simulink model "VFlexP"  (R2025a)
settings: Solver=ode23tb  StartTime=0.0  StopTime=40  FixedStep=5e-5
model workspace (MAT data in the model file):
  DCop_DCBUCK.op = opcond.OperatingPoint
  DCop_DCBUCK.op.Model_ = 'untitled4'
  DCop_DCBUCK.op.States_(1) = opcond.StatePoint
  DCop_DCBUCK.op.States_(1).Nx_ = 1
  DCop_DCBUCK.op.States_(1).Block_ = 'untitled4/DCBUCK/Integrator'
  DCop_DCBUCK.op.States_(1).x_ = 0.0993111458289
  DCop_DCBUCK.op.States_(2) = opcond.StatePoint
  DCop_DCBUCK.op.States_(2).Nx_ = 1
  DCop_DCBUCK.op.States_(2).Block_ = 'untitled4/DCBUCK/Integrator1'
  DCop_DCBUCK.op.States_(2).x_ = -1.0059432275
  DCop_DCBUCK.op_report = opcond.OperatingReport
  DCop_DCBUCK.op_report.Outputs_ = opcond.OutputReport
  DCop_DCBUCK.op_report.Outputs_.yspec_ = 0.0993111426985
  DCop_DCBUCK.op_report.Outputs_.Block_ = 'untitled4/out_trim1'
  DCop_DCBUCK.op_report.Outputs_.PortWidth_ = 1
  DCop_DCBUCK.op_report.Outputs_.PortNumber_ = NaN
  DCop_DCBUCK.op_report.Outputs_.y_ = 0.0993111458289
  DCop_DCBUCK.op_report.Outputs_.Known_ = 1
  DCop_DCBUCK.op_report.Outputs_.Min_ = -Inf
  DCop_DCBUCK.op_report.Outputs_.Max_ = Inf
  DCop_DCBUCK.op_report.TerminationString_ = 'Operating point specifications were successfully met.'
  DCop_DCBUCK.op_report.OptimizationOutput_.iterations = 1
  DCop_DCBUCK.op_report.OptimizationOutput_.funcCount = 6
  DCop_DCBUCK.op_report.OptimizationOutput_.constrviolation = 8.64996069397e-05
  DCop_DCBUCK.op_report.OptimizationOutput_.stepsize = 2.19887440386
  DCop_DCBUCK.op_report.OptimizationOutput_.algorithm = 'interior-point'
  DCop_DCBUCK.op_report.OptimizationOutput_.firstorderopt = 0
  DCop_DCBUCK.op_report.OptimizationOutput_.cgiterations = 0
  DCop_DCBUCK.op_report.OptimizationOutput_.message = 'Local minimum found that satisfies the constraints.
    | 
    | Optimization completed because the objective function is non-decreasing in 
    | feasible directions, to within the value of the optimality tolerance,
    | and constraints are satisfied to within the value of the constraint tolerance.
    | 
    | <stopping criteria details>
    | 
    | Optimization completed: The relative first-order optimality measure, 0.000000e+00,
    | is less than options.OptimalityTolerance = 1.000000e-06, and the relative maximum constraint
    | violation, 9.451558e-09, is less than options.ConstraintTolerance = 1.000000e-06.'
  DCop_DCBUCK.op_report.OptimizationOutput_.bestfeasible = []
  DCop_DCBUCK.op_report.Model_ = 'untitled4'
  DCop_DCBUCK.op_report.States_(1) = opcond.StateReport
  DCop_DCBUCK.op_report.States_(1).dx_ = 8.64996069397e-05
  DCop_DCBUCK.op_report.States_(1).Nx_ = 1
  DCop_DCBUCK.op_report.States_(1).Block_ = 'untitled4/DCBUCK/Integrator'
  DCop_DCBUCK.op_report.States_(1).x_ = 0.0993111458289
  DCop_DCBUCK.op_report.States_(1).SteadyState_ = 1
  DCop_DCBUCK.op_report.States_(1).dxMin_ = -Inf
  DCop_DCBUCK.op_report.States_(1).dxMax_ = Inf
  DCop_DCBUCK.op_report.States_(1).Known_ = 0
  DCop_DCBUCK.op_report.States_(1).Min_ = -Inf
  DCop_DCBUCK.op_report.States_(1).Max_ = Inf
  DCop_DCBUCK.op_report.States_(2) = opcond.StateReport
  DCop_DCBUCK.op_report.States_(2).dx_ = -1.77018447944e-06
  DCop_DCBUCK.op_report.States_(2).Nx_ = 1
  DCop_DCBUCK.op_report.States_(2).Block_ = 'untitled4/DCBUCK/Integrator1'
  DCop_DCBUCK.op_report.States_(2).x_ = -1.0059432275
  DCop_DCBUCK.op_report.States_(2).SteadyState_ = 1
  DCop_DCBUCK.op_report.States_(2).dxMin_ = -Inf
  DCop_DCBUCK.op_report.States_(2).dxMax_ = Inf
  DCop_DCBUCK.op_report.States_(2).Known_ = 0
  DCop_DCBUCK.op_report.States_(2).Min_ = -Inf
  DCop_DCBUCK.op_report.States_(2).Max_ = Inf
  Grid_CCVSC_idx = [2; 3; 4; 5; 6; 7; 8; 9; 10; 11; 12]
  Grid_CCVSCs = 1
  Grid_CCVSCs_buses = 1
  Grid_CCVSCs_toM = [0 1 0 0 0 0 0 0 0 0 0 0 ... (781 elements, 71x11)]
  Grid_C_Lines = [0.1 0.1 0.1 0.1]
  Grid_Cbuses = [0.05000002 0.10000002 0.10000002 0.10000002 0.05000002]
  Grid_DC.include = 1
  Grid_DC.Nbuses = 3
  Grid_DC.from = [1; 2]
  Grid_DC.to = [2; 3]
  Grid_DC.bus = [3; 4; 5]
  Grid_DC.v = [0.9920000006 0.9960000002 1]
  Grid_DC.Lines_toM : sparse (value not decoded)
  Grid_DC.Lines_fromM : sparse (value not decoded)
  Grid_DC.R_Lines = [0.01 0.01]
  Grid_DC.L_Lines = [0 0]
  Grid_DC.CbusDC = [0.0001; 0.0001; 0.0001]
  Grid_DC.i_branch = [-0.39999996  -0.39999996; -0.39999998  -0.39999998]
  Grid_DC.Rbus = [50000000; 50000000; 50000000]
  Grid_DC.DC_CCVSCs_toM = [0  0; 1  0; 0  0; 0  1; 0  0]
  Grid_DC.DC_CCVSCs_DC_toM = [1  0; 0  0; 0  1]
  Grid_DC.DC_CCVSCs_buses = [2; 4]
  Grid_DC.DC_CCVSCs_DC_buses = [1; 3]
  Grid_DC.DC_CCVSC_dparams.ratio = [1 1]
  Grid_DC.DC_CCVSC_dparams.type = [1 2]
  Grid_DC.DC_CCVSC_dparams.Rf = [0.0001 0.0002]
  Grid_DC.DC_CCVSC_dparams.Lf = [0.15 0.35]
  Grid_DC.DC_CCVSC_dparams.alpha1 = [0.0001 0.0001]
  Grid_DC.DC_CCVSC_dparams.alpha2 = [0.015 0.015]
  Grid_DC.DC_CCVSC_dparams.alpha3 = [0.2 0.02]
  Grid_DC.DC_CCVSC_dparams.Gsw = [0 0]
  Grid_DCop_DCBUCK.op = opcond.OperatingPoint
  Grid_DCop_DCBUCK.op.Model_ = 'untitled'
  Grid_DCop_DCBUCK.op.States_(1) = opcond.StatePoint
  Grid_DCop_DCBUCK.op.States_(1).Nx_ = 1
  Grid_DCop_DCBUCK.op.States_(1).Block_ = 'untitled/DCBUCK/Integrator'
  Grid_DCop_DCBUCK.op.States_(1).x_ = 0.297042066445
  Grid_DCop_DCBUCK.op.States_(2) = opcond.StatePoint
  Grid_DCop_DCBUCK.op.States_(2).Nx_ = 1
  Grid_DCop_DCBUCK.op.States_(2).Block_ = 'untitled/DCBUCK/Integrator1'
  Grid_DCop_DCBUCK.op.States_(2).x_ = -1.00698752155
  Grid_DCop_DCBUCK.op_report = opcond.OperatingReport
  Grid_DCop_DCBUCK.op_report.Outputs_ = opcond.OutputReport
  Grid_DCop_DCBUCK.op_report.Outputs_.yspec_ = 0.297042068743
  Grid_DCop_DCBUCK.op_report.Outputs_.Block_ = 'untitled/out_trim1'
  Grid_DCop_DCBUCK.op_report.Outputs_.PortWidth_ = 1
  Grid_DCop_DCBUCK.op_report.Outputs_.PortNumber_ = NaN
  Grid_DCop_DCBUCK.op_report.Outputs_.y_ = 0.297042066445
  Grid_DCop_DCBUCK.op_report.Outputs_.Known_ = 1
  Grid_DCop_DCBUCK.op_report.Outputs_.Min_ = -Inf
  Grid_DCop_DCBUCK.op_report.Outputs_.Max_ = Inf
  Grid_DCop_DCBUCK.op_report.TerminationString_ = 'Operating point specifications were successfully met.'
  Grid_DCop_DCBUCK.op_report.OptimizationOutput_.iterations = 1
  Grid_DCop_DCBUCK.op_report.OptimizationOutput_.funcCount = 6
  Grid_DCop_DCBUCK.op_report.OptimizationOutput_.constrviolation = 8.27288844959e-05
  Grid_DCop_DCBUCK.op_report.OptimizationOutput_.stepsize = 2.12653445023
  Grid_DCop_DCBUCK.op_report.OptimizationOutput_.algorithm = 'interior-point'
  Grid_DCop_DCBUCK.op_report.OptimizationOutput_.firstorderopt = 0
  Grid_DCop_DCBUCK.op_report.OptimizationOutput_.cgiterations = 0
  Grid_DCop_DCBUCK.op_report.OptimizationOutput_.message = 'Local minimum found that satisfies the constraints.
    | 
    | Optimization completed because the objective function is non-decreasing in 
    | feasible directions, to within the value of the optimality tolerance,
    | and constraints are satisfied to within the value of the constraint tolerance.
    | 
    | <stopping criteria details>
    | 
    | Optimization completed: The relative first-order optimality measure, 0.000000e+00,
    | is less than options.OptimalityTolerance = 1.000000e-06, and the relative maximum constraint
    | violation, 8.342696e-09, is less than options.ConstraintTolerance = 1.000000e-06.'
  Grid_DCop_DCBUCK.op_report.OptimizationOutput_.bestfeasible = []
  Grid_DCop_DCBUCK.op_report.Model_ = 'untitled'
  Grid_DCop_DCBUCK.op_report.States_(1) = opcond.StateReport
  Grid_DCop_DCBUCK.op_report.States_(1).dx_ = 8.27288844959e-05
  Grid_DCop_DCBUCK.op_report.States_(1).Nx_ = 1
  Grid_DCop_DCBUCK.op_report.States_(1).Block_ = 'untitled/DCBUCK/Integrator'
  Grid_DCop_DCBUCK.op_report.States_(1).x_ = 0.297042066445
  Grid_DCop_DCBUCK.op_report.States_(1).SteadyState_ = 1
  Grid_DCop_DCBUCK.op_report.States_(1).dxMin_ = -Inf
  Grid_DCop_DCBUCK.op_report.States_(1).dxMax_ = Inf
  Grid_DCop_DCBUCK.op_report.States_(1).Known_ = 0
  Grid_DCop_DCBUCK.op_report.States_(1).Min_ = -Inf
  Grid_DCop_DCBUCK.op_report.States_(1).Max_ = Inf
  Grid_DCop_DCBUCK.op_report.States_(2) = opcond.StateReport
  Grid_DCop_DCBUCK.op_report.States_(2).dx_ = 1.29998784019e-06
  Grid_DCop_DCBUCK.op_report.States_(2).Nx_ = 1
  Grid_DCop_DCBUCK.op_report.States_(2).Block_ = 'untitled/DCBUCK/Integrator1'
  Grid_DCop_DCBUCK.op_report.States_(2).x_ = -1.00698752155
  Grid_DCop_DCBUCK.op_report.States_(2).SteadyState_ = 1
  Grid_DCop_DCBUCK.op_report.States_(2).dxMin_ = -Inf
  Grid_DCop_DCBUCK.op_report.States_(2).dxMax_ = Inf
  Grid_DCop_DCBUCK.op_report.States_(2).Known_ = 0
  Grid_DCop_DCBUCK.op_report.States_(2).Min_ = -Inf
  Grid_DCop_DCBUCK.op_report.States_(2).Max_ = Inf
  Grid_DCop_DC_PES.op = opcond.OperatingPoint
  Grid_DCop_DC_PES.op.Model_ = 'untitled'
  Grid_DCop_DC_PES.op.States_(1) = opcond.StatePoint
  Grid_DCop_DC_PES.op.States_(1).Nx_ = 1
  Grid_DCop_DC_PES.op.States_(1).Block_ = 'untitled/DC_PES/Integrator'
  Grid_DCop_DC_PES.op.States_(1).x_ = 0.0833333466671
  Grid_DCop_DC_PES.op.States_(2) = opcond.StatePoint
  Grid_DCop_DC_PES.op.States_(2).Nx_ = 1
  Grid_DCop_DC_PES.op.States_(2).Block_ = 'untitled/DC_PES/Integrator1'
  Grid_DCop_DC_PES.op.States_(2).x_ = 0.166666684167
  Grid_DCop_DC_PES.op.States_(3) = opcond.StatePoint
  Grid_DCop_DC_PES.op.States_(3).Nx_ = 1
  Grid_DCop_DC_PES.op.States_(3).Block_ = 'untitled/DC_PES/Integrator2'
  Grid_DCop_DC_PES.op.States_(3).x_ = 0.0833333466671
  Grid_DCop_DC_PES.op.States_(4) = opcond.StatePoint
  Grid_DCop_DC_PES.op.States_(4).Nx_ = 1
  Grid_DCop_DC_PES.op.States_(4).Block_ = 'untitled/DC_PES/WOF_d/I'
  Grid_DCop_DC_PES.op.States_(4).x_ = 9.16666653332e-13
  Grid_DCop_DC_PES.op_report = opcond.OperatingReport
  Grid_DCop_DC_PES.op_report.Outputs_ = opcond.OutputReport
  Grid_DCop_DC_PES.op_report.Outputs_.yspec_ = 0.166666666667
  Grid_DCop_DC_PES.op_report.Outputs_.Block_ = 'untitled/out_trim1'
  Grid_DCop_DC_PES.op_report.Outputs_.PortWidth_ = 1
  Grid_DCop_DC_PES.op_report.Outputs_.PortNumber_ = NaN
  Grid_DCop_DC_PES.op_report.Outputs_.y_ = 0.166666684167
  Grid_DCop_DC_PES.op_report.Outputs_.Known_ = 1
  Grid_DCop_DC_PES.op_report.Outputs_.Min_ = -Inf
  Grid_DCop_DC_PES.op_report.Outputs_.Max_ = Inf
  Grid_DCop_DC_PES.op_report.TerminationString_ = 'Operating point specifications were successfully met.'
  Grid_DCop_DC_PES.op_report.OptimizationOutput_.iterations = 1
  Grid_DCop_DC_PES.op_report.OptimizationOutput_.funcCount = 10
  Grid_DCop_DC_PES.op_report.OptimizationOutput_.constrviolation = 1.74999997271e-08
  Grid_DCop_DC_PES.op_report.OptimizationOutput_.stepsize = 1.54110347542
  Grid_DCop_DC_PES.op_report.OptimizationOutput_.algorithm = 'interior-point'
  Grid_DCop_DC_PES.op_report.OptimizationOutput_.firstorderopt = 0
  Grid_DCop_DC_PES.op_report.OptimizationOutput_.cgiterations = 0
  Grid_DCop_DC_PES.op_report.OptimizationOutput_.message = 'Local minimum found that satisfies the constraints.
    | 
    | Optimization completed because the objective function is non-decreasing in 
    | feasible directions, to within the value of the optimality tolerance,
    | and constraints are satisfied to within the value of the constraint tolerance.
    | 
    | <stopping criteria details>
    | 
    | Optimization completed: The relative first-order optimality measure, 0.000000e+00,
    | is less than options.OptimalityTolerance = 1.000000e-06, and the relative maximum constraint
    | violation, 1.750000e-08, is less than options.ConstraintTolerance = 1.000000e-06.'
  Grid_DCop_DC_PES.op_report.OptimizationOutput_.bestfeasible.x = [0.166666684167; 9.16666653332e-13; 0.0833333466671; 0.0833333466671]
  Grid_DCop_DC_PES.op_report.OptimizationOutput_.bestfeasible.fval = 0
  Grid_DCop_DC_PES.op_report.OptimizationOutput_.bestfeasible.constrviolation = 1.74999997271e-08
  Grid_DCop_DC_PES.op_report.OptimizationOutput_.bestfeasible.firstorderopt = 0
  Grid_DCop_DC_PES.op_report.Model_ = 'untitled'
  Grid_DCop_DC_PES.op_report.States_(1) = opcond.StateReport
  Grid_DCop_DC_PES.op_report.States_(1).Nx_ = 1
  Grid_DCop_DC_PES.op_report.States_(1).Block_ = 'untitled/DC_PES/Integrator'
  Grid_DCop_DC_PES.op_report.States_(1).x_ = 0.0833333466671
  Grid_DCop_DC_PES.op_report.States_(1).SteadyState_ = 1
  Grid_DCop_DC_PES.op_report.States_(1).dxMin_ = -Inf
  Grid_DCop_DC_PES.op_report.States_(1).dxMax_ = Inf
  Grid_DCop_DC_PES.op_report.States_(1).Known_ = 0
  Grid_DCop_DC_PES.op_report.States_(1).Min_ = -Inf
  Grid_DCop_DC_PES.op_report.States_(1).Max_ = Inf
  Grid_DCop_DC_PES.op_report.States_(2) = opcond.StateReport
  Grid_DCop_DC_PES.op_report.States_(2).dx_ = 9.16666659245e-09
  Grid_DCop_DC_PES.op_report.States_(2).Nx_ = 1
  Grid_DCop_DC_PES.op_report.States_(2).Block_ = 'untitled/DC_PES/Integrator1'
  Grid_DCop_DC_PES.op_report.States_(2).x_ = 0.166666684167
  Grid_DCop_DC_PES.op_report.States_(2).SteadyState_ = 1
  Grid_DCop_DC_PES.op_report.States_(2).dxMin_ = -Inf
  Grid_DCop_DC_PES.op_report.States_(2).dxMax_ = Inf
  Grid_DCop_DC_PES.op_report.States_(2).Known_ = 0
  Grid_DCop_DC_PES.op_report.States_(2).Min_ = -Inf
  Grid_DCop_DC_PES.op_report.States_(2).Max_ = Inf
  Grid_DCop_DC_PES.op_report.States_(3) = opcond.StateReport
  Grid_DCop_DC_PES.op_report.States_(3).Nx_ = 1
  Grid_DCop_DC_PES.op_report.States_(3).Block_ = 'untitled/DC_PES/Integrator2'
  Grid_DCop_DC_PES.op_report.States_(3).x_ = 0.0833333466671
  Grid_DCop_DC_PES.op_report.States_(3).SteadyState_ = 1
  Grid_DCop_DC_PES.op_report.States_(3).dxMin_ = -Inf
  Grid_DCop_DC_PES.op_report.States_(3).dxMax_ = Inf
  Grid_DCop_DC_PES.op_report.States_(3).Known_ = 0
  Grid_DCop_DC_PES.op_report.States_(3).Min_ = -Inf
  Grid_DCop_DC_PES.op_report.States_(3).Max_ = Inf
  Grid_DCop_DC_PES.op_report.States_(4) = opcond.StateReport
  Grid_DCop_DC_PES.op_report.States_(4).dx_ = -9.16666653332e-11
  Grid_DCop_DC_PES.op_report.States_(4).Nx_ = 1
  Grid_DCop_DC_PES.op_report.States_(4).Block_ = 'untitled/DC_PES/WOF_d/I'
  Grid_DCop_DC_PES.op_report.States_(4).x_ = 9.16666653332e-13
  Grid_DCop_DC_PES.op_report.States_(4).SteadyState_ = 1
  Grid_DCop_DC_PES.op_report.States_(4).dxMin_ = -Inf
  Grid_DCop_DC_PES.op_report.States_(4).dxMax_ = Inf
  Grid_DCop_DC_PES.op_report.States_(4).Known_ = 0
  Grid_DCop_DC_PES.op_report.States_(4).Min_ = -Inf
  Grid_DCop_DC_PES.op_report.States_(4).Max_ = Inf
  Grid_DFIGs = 1
  Grid_DFIGs_buses = 1
  Grid_DGs = ["MGES"; "MGES"; "MGES"]
  Grid_From_buses = [1 2 4 4]
  Grid_GFls = 1
  Grid_GFls_buses = 1
  Grid_GFr_idx = [1; 2; 3]
  Grid_GFrs = 1
  Grid_GFrs_buses = 1
  Grid_GFrs_toM = [1 0 0 0 0 0 0 0 0 1 0 0 ... (15 elements, 5x3)]
  Grid_IG_idx = 1
  Grid_IGs = 1
  Grid_IGs_buses = 1
  Grid_IGs_toM = [1; 0]
  Grid_L_Lines = [0.5 0.5 0.5 0.5]
  Grid_L_Loads = [0.000959999944704 0.000156249997559 0.00154855477548]
  Grid_Lines_fromM : object (value not decoded)
  Grid_Lines_toM : object (value not decoded)
  Grid_Load_buses = [2; 3; 4]
  Grid_Load_busesDC = []
  Grid_MGES_idx = [1; 2; 3]
  Grid_MGESs = 1
  Grid_MGESs_buses = [1; 5; 3]
  Grid_MGESs_toM = [1 0 0 0 0 0 0 0 0 1 0 0 ... (15 elements, 5x3)]
  Grid_MSGs = 1
  Grid_MSGs_buses = 1
  Grid_Nbuses = 5
  Grid_PQ_gen = [3; 2; 2]
  Grid_Ploads = [1250 4000 1250]
  Grid_PloadsDC = []
  Grid_Ps_lf = [0.274439537683 0.78 0.3]
  Grid_Qloads = [0.3 0.5 0.5]
  Grid_Qs_lf = [-0.0366071562958 0.126505596722 -0.0162964024532]
  Grid_R_Lines = [0.01 0.01 0.01 0.01]
  Grid_R_Loads = [3.9999997696 1.24999998047 3.8713869387]
  Grid_R_Loads_DC = 0
  Grid_Rcf = [50000000 50000000 50000000 50000000 50000000]
  Grid_SCs = 1
  Grid_SCs_buses = 1
  Grid_SG_idx = 1
  Grid_SGs = 1
  Grid_SGs_buses = 1
  Grid_SGs_toM = [1; 0]
  Grid_To_buses = [2 3 3 5]
  Grid_VCVSC_idx = [1; 2; 3; 4; 5; 6; 7; 8; 9; 10; 11; 12]
  Grid_VCVSCs = 1
  Grid_VCVSCs_buses = [1; 2; 3; 6; 8; 9; 12; 58; 59; 60; 63; 65]
  Grid_VCVSCs_toM = [1 0 0 0 0 0 0 0 0 0 0 0 ... (852 elements, 71x12)]
  Grid_VSM_idx = [1; 2; 3]
  Grid_VSMs = 1
  Grid_VSMs_buses = 1
  Grid_VSMs_toM = [1 0 0 0 0 0 0 0 0 1 0 0 ... (15 elements, 5x3)]
  Grid_admitt_matrix = [2.15353135314-19.7953135314i  -1.9801980198+19.801980198i; -1.9801980198+19.801980198i  2.15353135314-19.7953135314i]
  Grid_admitt_matrix_noloads = [1.98686468647-19.7953135314i  -1.9801980198+19.801980198i; -1.9801980198+19.801980198i  1.98686468647-19.7953135314i]
  Grid_bus = [1; 2; 6; 7; 8]
  Grid_busDC_complexity = [1 1 1]
  Grid_busDC_complexity_PF = [2 2 2]
  Grid_bus_complexity = [1 1 1 1 1]
  Grid_bus_complexity_PF = [1 1 1 1 1]
  Grid_buses_lf = [1; 5; 3]
  Grid_conductance_matrix = [100.00000002  -100  0; -100  200.00000002  -100; 0  -100  100.00000002]
  Grid_conductance_matrix_noloads = [100.00000002  -100  0; -100  200.00000002  -100; 0  -100  100.00000002]
  Grid_fref.areas = 1
  Grid_fref.ref_units = 1
  Grid_fref.Fb_units = [1 1 1]
  Grid_fref.buses = [1 1 1 1 1]
  Grid_fref.lines = [1 1 1 1]
  Grid_fref.loads = [1 1 1]
  Grid_fref.MGES = [1 1 1]
  Grid_fref.DC_CCVSC = [1 1]
  Grid_gen_static_params.mBase = [1500; 5000; 1500]
  Grid_iPs_lf = [3.64378984326 1.28205128205 3.33333333333]
  Grid_iQs_lf = [-27.3170631425 7.90478860943 -61.3632366329]
  Grid_iadmitt_matrix = [2.88165849328-0.0982918688642i  2.87905051706-0.123273862303i; 2.87905051706-0.123273862303i  2.88165849328-0.0982918688642i]
  Grid_iadmitt_matrix_noloads = [37.5012524798-37.4874983544i  37.4987475202-37.5125016456i; 37.4987475202-37.5125016456i  37.5012524798-37.4874983544i]
  Grid_iconductance_matrix = [16666671.4556  16666671.4489  16666671.4456; 16666671.4489  16666671.4522  16666671.4489; 16666671.4456  16666671.4489  16666671.4556]
  Grid_iconductance_matrix_noloads = [16666671.4556  16666671.4489  16666671.4456; 16666671.4489  16666671.4522  16666671.4489; 16666671.4456  16666671.4489  16666671.4556]
  Grid_init_OK_bool = 1
  Grid_intconv_PF.include = 1
  Grid_intconv_PF.vmod = [1 0.983792096676]
  Grid_intconv_PF.vangle = [-7.87925069062 -15.713681382]
  Grid_intconv_PF.P = [-0.364233596582 0.409865171394]
  Grid_intconv_PF.Q = [0.0454812254751 -0.0157475749063]
  Grid_intconv_PF.from = [1 2 3 4 7 7 3 5]
  Grid_intconv_PF.to = [2 6 4 5 6 8 2 7]
  Grid_lf_op.op_report.Outputs(1).y = [0.274439537683 0.78 0.3]
  Grid_lf_op.op_report.Outputs(2).y = [-0.0366071562958 0.126505596722 -0.0162964024532]
  Grid_lf_op.op_report.Outputs(3).y = [0.274439517683 0.380129105768 0.119782089106 -0.796402881523]
  Grid_lf_op.op_report.Outputs(4).y = [-0.0133928637042 -0.0829973268525 -0.00113579444539 0.0727781000897]
  Grid_lf_op.op_report.Outputs(5).y = [0.247631568093 0.756174742749 0.244594049574]
  Grid_lf_op.op_report.Outputs(6).y = [-0.0343308911015 -0.261150853778 -0.068920904761]
  Grid_lf_op.op_report.Outputs(7).y = [1 0.990559172971 0.945259218487 0.947024936601 0.991378015461]
  Grid_lf_op.op_report.Outputs(8).y = [0 -0.137085830204 -0.32632040982 -0.266440723211 0.131032936549]
  Grid_lineDC_complexity = [1 1]
  Grid_lineDC_complexity_PF = [2 2]
  Grid_line_complexity = [1 1 1 1]
  Grid_line_complexity_PF = [3 3 3 3]
  Grid_loadDC_complexity = []
  Grid_loadDC_complexity_PF = []
  Grid_load_complexity = [3 3 3]
  Grid_load_complexity_PF = [4 4 4]
  Grid_opDC_CCVSC.P = [0.364233596582 -0.409865171394]
  Grid_opDC_CCVSC.Q = [-0.0454812254751 0.0157475749063]
  Grid_opDC_CCVSC.id_out = [0.364233596582 -0.416617670318]
  Grid_opDC_CCVSC.iq_out = [0.0454812254751 -0.0160070150588]
  Grid_opDC_CCVSC.PId = [3.64233596583e-05 -8.33235340636e-05]
  Grid_opDC_CCVSC.PIq = [4.5481225475e-06 -3.20140301172e-06]
  Grid_opDC_CCVSC.frame = [-0.137518867141 -0.274255477725]
  Grid_opDC_VSM.P = 0.158097434546
  Grid_opDC_VSM.Q = 0.34570155769
  Grid_opDC_VSM.id_out = 0.15491365585
  Grid_opDC_VSM.iq_out = -0.347139921401
  Grid_opDC_VSM.frame = -0.00374877829395
  Grid_opDC_VSM.vd_c = 1.01233482292
  Grid_opDC_VSM.vq_c = 4.33680868994e-19
  Grid_opDC_VSM.id_l = 0.156214927213
  Grid_opDC_VSM.iq_l = -0.245323264284
  Grid_opDC_VSM.id_in = 0.000109431280071
  Grid_opDC_VSM.iq_in = -0.000245220253528
  Grid_opDC_VSM.PIid = 0.000367835001532
  Grid_opDC_VSM.PIiq = -0.000577655957108
  Grid_opDC_VSM.PIvd = 7.90886580402e-07
  Grid_opDC_VSM.PIvq = -1.08420217249e-17
  Grid_opDC_VSM.IP = 0
  Grid_opDC_VSM.iv = 0.0123348229164
  Grid_opGFr.Pd = [0.59436535015 0.0005 0.0005]
  Grid_opGFr.Qd = [0.0279865855357 -0.0637915242449 0.286980765211]
  Grid_opGFr.id_out = [0.59436535015 0.0567408703424 -0.212812144187]
  Grid_opGFr.iq_out = [-0.0279865855357 0.0291561691289 -0.192533635731]
  Grid_opGFr.frame = [0.00591043094825 -1.08822527402 -0.837407617783]
  Grid_opGFr.vd_c = [1.00089171333 0.999362587125 1.00287034729]
  Grid_opGFr.vq_c = [0 0 -5.55111512313e-17]
  Grid_opGFr.iV = [0.000891713326809 -0.000637412874803 0.0028703472949]
  Grid_opGFr.v = [1.00089171333 0.999362587125 1.00287034729]
  Grid_opGFr.IntConnect = [5 5 5]
  Grid_opGFr.id_l = [0.594190557714 0.000505390476543 0.000581694293892]
  Grid_opGFr.iq_l = [0.068590139719 0.163727748389 -0.18669357855]
  Grid_opGFr.PIid = [0.00594190557714 5.05390476543e-06 5.81694293892e-06]
  Grid_opGFr.PIiq = [0.00068590139719 0.00163727748389 -0.0018669357855]
  Grid_opGFr.PIvd = [1.00089171329e-05 9.99362587125e-06 1.00287034729e-05]
  Grid_opGFr.PIvq = [0 0 0]
  Grid_opVCVSC.Pd = 0
  Grid_opVCVSC.Qd = 0
  Grid_opVCVSC.id_out = [4.77012824674 0.000252372172029 0.387206076232 -0.00669815177796 4.43044477222 -0.00888398142826 2.79473009232 2.18798980312 0.322264460806 -0.0632019138679 -0.0604985051331 -0.0462539180443]
  Grid_opVCVSC.iq_out = [-1.25997186372 0.0149684790164 -0.231751502643 -0.0494644982143 -0.911066731256 -0.0589472249505 -1.80353640382 0.162268294537 -1.0981777606 -0.338765693762 -0.298705341855 -0.251695536875]
  Grid_opVCVSC.frame = [0.0438933282651 -0.0168438196467 -0.0841666076082 -0.134645533542 -0.017373173296 -0.149645793269 -0.137562101317 0.0572176344752 -0.0529798109092 -0.184784853699 -0.200116593784 -0.181975782571]
  Grid_opVCVSC.vd_c = [1.0583892424 1.00985029405 0.987381572831 0.980499160746 1.0168380704 0.980596131031 1.0316409122 1.06159711208 1.05617213999 1.01344616766 1.07304774652 1.09255913271]
  Grid_opVCVSC.vq_c = [6.93889390391e-18 3.46944695195e-18 0 2.77555756156e-17 0 -2.77555756156e-17 0 -6.93889390391e-18 6.93889390391e-18 -2.77555756156e-17 0 2.77555756156e-17]
  Grid_opVCVSC.iV = [0.0183892424009 -0.000149705952964 0.00238157283064 0.00049916074618 0.0118380704031 0.000596131030837 0.0166409121976 0.00159711208293 0.0111721399885 0.00344616765999 0.00304774652066 0.00255913270857]
  Grid_opVCVSC.v = [1.0583892424 1.00985029405 0.987381572831 0.980499160746 1.0168380704 0.980596131031 1.0316409122 1.06159711208 1.05617213999 1.01344616766 1.07304774652 1.09255913271]
  Grid_opVCVSC.id_l = [4.71024831855 1.231783245e-06 0.405319101793 3.52165566611e-06 4.44560451561 4.60461660484e-06 3.01564651745 2.19368980083 0.379967383234 0.000118194487427 8.76348532929e-05 6.10344572474e-05]
  Grid_opVCVSC.iq_l = [-1.36222896789 0.115955635796 -0.0996416062474 0.0481339685791 -0.732278422455 0.0384466913306 -1.30009716484 0.143039154495 -0.973954167095 -0.243266270257 -0.197465537031 -0.146654353471]
  Grid_opVCVSC.PIid = [0.000135655151574 3.5475357456e-11 1.16731901316e-05 1.01423683184e-10 0.00012803341005 1.32612958219e-10 8.68506197027e-05 6.31782662639e-05 1.09430606371e-05 3.40400123789e-09 2.52388377483e-09 1.75779236873e-09]
  Grid_opVCVSC.PIiq = [-3.92321942752e-05 3.33952231093e-06 -2.86967825993e-06 1.38625829508e-06 -2.10896185667e-05 1.10726471032e-06 -3.74427983473e-05 4.11952764945e-06 -2.80498800123e-05 -7.00606858342e-06 -5.68700746649e-06 -4.22364537998e-06]
  Grid_opVCVSC.PIvd = [3.67496264593e-05 3.50642463211e-05 3.42840823902e-05 3.40451097481e-05 3.53068774525e-05 3.40484767719e-05 3.58208650088e-05 3.68610108331e-05 3.66726437489e-05 3.51891030437e-05 3.72586023097e-05 3.79360809968e-05]
  Grid_opVCVSC.PIvq = [-3.85494105773e-15 0 0 0 4.81867632216e-16 0 -2.40933816108e-15 4.81867632216e-16 0 0 -4.81867632216e-16 -4.81867632216e-16]
  Grid_op_CCVSC.op = opcond.OperatingPoint
  Grid_op_CCVSC.op.Model_ = 'untitled'
  Grid_op_CCVSC.op.States_(1) = opcond.StatePoint
  Grid_op_CCVSC.op.States_(1).Nx_ = 11
  Grid_op_CCVSC.op.States_(1).Block_ = 'untitled/CCVSC/LPF/I'
  Grid_op_CCVSC.op.States_(1).x_ = [1.009861943; 0.981291076401; 0.971352962827; 1.00322239915; 0.969168759309; 1.00101830201; 1.05929040967; 1.04339572399; 0.992934596599; 1.04879026715; 1.07220457445]
  Grid_op_CCVSC.op.States_(2) = opcond.StatePoint
  Grid_op_CCVSC.op.States_(2).Nx_ = 11
  Grid_op_CCVSC.op.States_(2).Block_ = 'untitled/CCVSC/LPF1/I'
  Grid_op_CCVSC.op.States_(2).x_ = [-0.0166989844806; -0.085398033397; -0.129897735513; -0.0597487458922; -0.14529940151; -0.167892796173; 0.038779556309; -0.0578823653869; -0.184880740706; -0.211988173785; -0.196156450928]
  Grid_op_CCVSC.op.States_(3) = opcond.StatePoint
  Grid_op_CCVSC.op.States_(3).Nx_ = 11
  Grid_op_CCVSC.op.States_(3).Block_ = 'untitled/CCVSC/LPF2/I'
  Grid_op_CCVSC.op.States_(3).x_ = [1.009861943; 0.981291076401; 0.971352962827; 1.00322239915; 0.969168759309; 1.00101830201; 1.05929040967; 1.04339572399; 0.992934596599; 1.04879026715; 1.07220457445]
  Grid_op_CCVSC.op.States_(4) = opcond.StatePoint
  Grid_op_CCVSC.op.States_(4).Nx_ = 11
  Grid_op_CCVSC.op.States_(4).Block_ = 'untitled/CCVSC/LPF3/I'
  Grid_op_CCVSC.op.States_(4).x_ = [-0.0166989844806; -0.085398033397; -0.129897735513; -0.0597487458926; -0.14529940151; -0.167892796174; 0.0387795563087; -0.0578823653869; -0.184880740706; -0.211988173785; -0.196156450928]
  Grid_op_CCVSC.op.States_(5) = opcond.StatePoint
  Grid_op_CCVSC.op.States_(5).Nx_ = 11
  Grid_op_CCVSC.op.States_(5).Block_ = 'untitled/CCVSC/P'
  Grid_op_CCVSC.op.States_(5).x_ = [1.01727038409e-18; 0.400000000001; -1.80456749167e-13; 4.5000000022; 3.15175961175e-13; 3.10000001288; 2.32400000036; 0.400000000095; -1.95503794004e-12; -3.47571023681e-11; 9.07830100881e-12]
  Grid_op_CCVSC.op.States_(6) = opcond.StatePoint
  Grid_op_CCVSC.op.States_(6).Nx_ = 11
  Grid_op_CCVSC.op.States_(6).Block_ = 'untitled/CCVSC/PLL/dynamic/PLL/I'
  Grid_op_CCVSC.op.States_(6).x_ = [1; 1; 1; 0.999999999991; 1; 0.999999999962; 1; 1; 1; 1; 1]
  Grid_op_CCVSC.op.States_(7) = opcond.StatePoint
  Grid_op_CCVSC.op.States_(7).Nx_ = 11
  Grid_op_CCVSC.op.States_(7).Block_ = 'untitled/CCVSC/PLL/dynamic/frame'
  Grid_op_CCVSC.op.States_(7).x_ = [-0.0165344013704; -0.0868074935304; -0.132939939029; -0.0594865631615; -0.148813342999; -0.166175316605; 0.0365926525094; -0.0554181853462; -0.184088222665; -0.199439311658; -0.180945834503]
  Grid_op_CCVSC.op.States_(8) = opcond.StatePoint
  Grid_op_CCVSC.op.States_(8).Nx_ = 11
  Grid_op_CCVSC.op.States_(8).Block_ = 'untitled/CCVSC/Q'
  Grid_op_CCVSC.op.States_(8).x_ = [-0.015862822257; 0.120252486258; 0.0522438711347; 0.647307088531; 0.0546742450618; 1.36800880468; -0.0931237077542; 1.06159295924; 0.342624354062; 0.31755952052; 0.276277445204]
  Grid_op_CCVSC.op_report = opcond.OperatingReport
  Grid_op_CCVSC.op_report.Outputs_(1) = opcond.OutputReport
  Grid_op_CCVSC.op_report.Outputs_(1).yspec_ = [0.000259673583656; 0.393977793367; -0.0070661813362; 4.43140001829; -0.00827169417353; 2.7891744299; 2.18777108046; 0.325918162006; -0.0620965046483; -0.05879890244; -0.0456136713835]
  Grid_op_CCVSC.op_report.Outputs_(1).Block_ = 'untitled/out_trim1'
  Grid_op_CCVSC.op_report.Outputs_(1).PortWidth_ = 11
  Grid_op_CCVSC.op_report.Outputs_(1).PortNumber_ = NaN
  Grid_op_CCVSC.op_report.Outputs_(1).y_ = [0.000259673583656; 0.393977793229; -0.00706618133531; 4.43139980848; -0.00827169417363; 2.78917339713; 2.18777105686; 0.325918157997; -0.0620965045362; -0.0587989014357; -0.0456136713993]
  Grid_op_CCVSC.op_report.Outputs_(1).Known_ = [1; 1; 1; 1; 1; 1; 1; 1; 1; 1; 1]
  Grid_op_CCVSC.op_report.Outputs_(1).Min_ = [-Inf; -Inf; -Inf; -Inf; -Inf; -Inf; -Inf; -Inf; -Inf; -Inf; -Inf]
  Grid_op_CCVSC.op_report.Outputs_(1).Max_ = [Inf; Inf; Inf; Inf; Inf; Inf; Inf; Inf; Inf; Inf; Inf]
  Grid_op_CCVSC.op_report.Outputs_(2) = opcond.OutputReport
  Grid_op_CCVSC.op_report.Outputs_(2).yspec_ = [0.0157036177884; -0.156831564843; -0.0528396907676; -0.909148054024; -0.0551734384103; -1.8344231967; 0.16800352209; -1.03552070385; -0.3335002201; -0.290901679261; -0.24932744737]
  Grid_op_CCVSC.op_report.Outputs_(2).Block_ = 'untitled/out_trim2'
  Grid_op_CCVSC.op_report.Outputs_(2).PortWidth_ = 11
  Grid_op_CCVSC.op_report.Outputs_(2).PortNumber_ = NaN
  Grid_op_CCVSC.op_report.Outputs_(2).y_ = [0.0157036177884; -0.156831564765; -0.0528396907661; -0.909148031788; -0.0551734384082; -1.83442292878; 0.168003502174; -1.03552070255; -0.333500219896; -0.29090167819; -0.249327447093]
  Grid_op_CCVSC.op_report.Outputs_(2).Known_ = [1; 1; 1; 1; 1; 1; 1; 1; 1; 1; 1]
  Grid_op_CCVSC.op_report.Outputs_(2).Min_ = [-Inf; -Inf; -Inf; -Inf; -Inf; -Inf; -Inf; -Inf; -Inf; -Inf; -Inf]
  Grid_op_CCVSC.op_report.Outputs_(2).Max_ = [Inf; Inf; Inf; Inf; Inf; Inf; Inf; Inf; Inf; Inf; Inf]
  Grid_op_CCVSC.op_report.TerminationString_ = 'Operating point specifications were successfully met.'
  Grid_op_CCVSC.op_report.OptimizationOutput_.iterations = 3
  Grid_op_CCVSC.op_report.OptimizationOutput_.funcCount = 356
  Grid_op_CCVSC.op_report.OptimizationOutput_.constrviolation = 2.89733602665e-05
  Grid_op_CCVSC.op_report.OptimizationOutput_.stepsize = 8.75730946062e-07
  Grid_op_CCVSC.op_report.OptimizationOutput_.algorithm = 'interior-point'
  Grid_op_CCVSC.op_report.OptimizationOutput_.firstorderopt = 0
  Grid_op_CCVSC.op_report.OptimizationOutput_.cgiterations = 0
  Grid_op_CCVSC.op_report.OptimizationOutput_.message = 'Local minimum found that satisfies the constraints.
    | 
    | Optimization completed because the objective function is non-decreasing in 
    | feasible directions, to within the value of the optimality tolerance,
    | and constraints are satisfied to within the value of the constraint tolerance.
    | 
    | <stopping criteria details>
    | 
    | Optimization completed: The relative first-order optimality measure, 0.000000e+00,
    | is less than options.OptimalityTolerance = 1.000000e-06, and the relative maximum constraint
    | violation, 6.438525e-07, is less than options.ConstraintTolerance = 1.000000e-06.'
  Grid_op_CCVSC.op_report.OptimizationOutput_.bestfeasible = []
  Grid_op_CCVSC.op_report.Model_ = 'untitled'
  Grid_op_CCVSC.op_report.States_(1) = opcond.StateReport
  Grid_op_CCVSC.op_report.States_(1).dx_ = [0; -8.881784197e-14; 3.33066907388e-14; 2.35367281221e-12; 6.66133814775e-14; -9.1748830755e-11; 8.881784197e-13; -6.12843109593e-12; 2.33146835171e-13; 1.04360964315e-12; -2.22044604925e-14]
  Grid_op_CCVSC.op_report.States_(1).Nx_ = 11
  Grid_op_CCVSC.op_report.States_(1).Block_ = 'untitled/CCVSC/LPF/I'
  Grid_op_CCVSC.op_report.States_(1).x_ = [1.009861943; 0.981291076401; 0.971352962827; 1.00322239915; 0.969168759309; 1.00101830201; 1.05929040967; 1.04339572399; 0.992934596599; 1.04879026715; 1.07220457445]
  Grid_op_CCVSC.op_report.States_(1).SteadyState_ = [1; 1; 1; 1; 1; 1; 1; 1; 1; 1; 1]
  Grid_op_CCVSC.op_report.States_(1).dxMin_ = [-Inf; -Inf; -Inf; -Inf; -Inf; -Inf; -Inf; -Inf; -Inf; -Inf; -Inf]
  Grid_op_CCVSC.op_report.States_(1).dxMax_ = [Inf; Inf; Inf; Inf; Inf; Inf; Inf; Inf; Inf; Inf; Inf]
  Grid_op_CCVSC.op_report.States_(1).Known_ = [0; 0; 0; 0; 0; 0; 0; 0; 0; 0; 0]
  Grid_op_CCVSC.op_report.States_(1).Min_ = [-Inf; -Inf; -Inf; -Inf; -Inf; -Inf; -Inf; -Inf; -Inf; -Inf; -Inf]
  Grid_op_CCVSC.op_report.States_(1).Max_ = [Inf; Inf; Inf; Inf; Inf; Inf; Inf; Inf; Inf; Inf; Inf]
  Grid_op_CCVSC.op_report.States_(2) = opcond.StateReport
  Grid_op_CCVSC.op_report.States_(2).dx_ = [0; 3.85802501057e-13; 3.80251385934e-13; -3.1668417888e-11; 4.27435864481e-13; -1.02551300785e-10; -2.89226975703e-11; 5.26662047307e-13; -9.99200722163e-14; -2.40363284831e-12; -1.34614541736e-12]
  Grid_op_CCVSC.op_report.States_(2).Nx_ = 11
  Grid_op_CCVSC.op_report.States_(2).Block_ = 'untitled/CCVSC/LPF1/I'
  Grid_op_CCVSC.op_report.States_(2).x_ = [-0.0166989844806; -0.085398033397; -0.129897735513; -0.0597487458922; -0.14529940151; -0.167892796173; 0.038779556309; -0.0578823653869; -0.184880740706; -0.211988173785; -0.196156450928]
  Grid_op_CCVSC.op_report.States_(2).SteadyState_ = [1; 1; 1; 1; 1; 1; 1; 1; 1; 1; 1]
  Grid_op_CCVSC.op_report.States_(2).dxMin_ = [-Inf; -Inf; -Inf; -Inf; -Inf; -Inf; -Inf; -Inf; -Inf; -Inf; -Inf]
  Grid_op_CCVSC.op_report.States_(2).dxMax_ = [Inf; Inf; Inf; Inf; Inf; Inf; Inf; Inf; Inf; Inf; Inf]
  Grid_op_CCVSC.op_report.States_(2).Known_ = [0; 0; 0; 0; 0; 0; 0; 0; 0; 0; 0]
  Grid_op_CCVSC.op_report.States_(2).Min_ = [-Inf; -Inf; -Inf; -Inf; -Inf; -Inf; -Inf; -Inf; -Inf; -Inf; -Inf]
  Grid_op_CCVSC.op_report.States_(2).Max_ = [Inf; Inf; Inf; Inf; Inf; Inf; Inf; Inf; Inf; Inf; Inf]
  Grid_op_CCVSC.op_report.States_(3) = opcond.StateReport
  Grid_op_CCVSC.op_report.States_(3).dx_ = [0; -3.7627989613e-08; -4.49945636305e-09; -4.6817306476e-06; -4.84622342256e-09; -2.89733602665e-05; -1.25802135376e-06; -2.23016383138e-07; -7.25810522795e-08; -5.29354471368e-07; -1.1638969788e-07]
  Grid_op_CCVSC.op_report.States_(3).Nx_ = 11
  Grid_op_CCVSC.op_report.States_(3).Block_ = 'untitled/CCVSC/LPF2/I'
  Grid_op_CCVSC.op_report.States_(3).x_ = [1.009861943; 0.981291076401; 0.971352962827; 1.00322239915; 0.969168759309; 1.00101830201; 1.05929040967; 1.04339572399; 0.992934596599; 1.04879026715; 1.07220457445]
  Grid_op_CCVSC.op_report.States_(3).SteadyState_ = [1; 1; 1; 1; 1; 1; 1; 1; 1; 1; 1]
  Grid_op_CCVSC.op_report.States_(3).dxMin_ = [-Inf; -Inf; -Inf; -Inf; -Inf; -Inf; -Inf; -Inf; -Inf; -Inf; -Inf]
  Grid_op_CCVSC.op_report.States_(3).dxMax_ = [Inf; Inf; Inf; Inf; Inf; Inf; Inf; Inf; Inf; Inf; Inf]
  Grid_op_CCVSC.op_report.States_(3).Known_ = [0; 0; 0; 0; 0; 0; 0; 0; 0; 0; 0]
  Grid_op_CCVSC.op_report.States_(3).Min_ = [-Inf; -Inf; -Inf; -Inf; -Inf; -Inf; -Inf; -Inf; -Inf; -Inf; -Inf]
  Grid_op_CCVSC.op_report.States_(3).Max_ = [Inf; Inf; Inf; Inf; Inf; Inf; Inf; Inf; Inf; Inf; Inf]
  Grid_op_CCVSC.op_report.States_(4) = opcond.StateReport
  Grid_op_CCVSC.op_report.States_(4).dx_ = [0; -3.13662568141e-09; -1.01869901403e-09; 7.20071362953e-07; 2.0284746105e-09; 1.545790487e-05; 8.24665298549e-07; 3.50140891281e-07; -9.12854514201e-09; -1.88931087441e-07; 5.35036820404e-08]
  Grid_op_CCVSC.op_report.States_(4).Nx_ = 11
  Grid_op_CCVSC.op_report.States_(4).Block_ = 'untitled/CCVSC/LPF3/I'
  Grid_op_CCVSC.op_report.States_(4).x_ = [-0.0166989844806; -0.085398033397; -0.129897735513; -0.0597487458926; -0.14529940151; -0.167892796174; 0.0387795563087; -0.0578823653869; -0.184880740706; -0.211988173785; -0.196156450928]
  Grid_op_CCVSC.op_report.States_(4).SteadyState_ = [1; 1; 1; 1; 1; 1; 1; 1; 1; 1; 1]
  Grid_op_CCVSC.op_report.States_(4).dxMin_ = [-Inf; -Inf; -Inf; -Inf; -Inf; -Inf; -Inf; -Inf; -Inf; -Inf; -Inf]
  Grid_op_CCVSC.op_report.States_(4).dxMax_ = [Inf; Inf; Inf; Inf; Inf; Inf; Inf; Inf; Inf; Inf; Inf]
  Grid_op_CCVSC.op_report.States_(4).Known_ = [0; 0; 0; 0; 0; 0; 0; 0; 0; 0; 0]
  Grid_op_CCVSC.op_report.States_(4).Min_ = [-Inf; -Inf; -Inf; -Inf; -Inf; -Inf; -Inf; -Inf; -Inf; -Inf; -Inf]
  Grid_op_CCVSC.op_report.States_(4).Max_ = [Inf; Inf; Inf; Inf; Inf; Inf; Inf; Inf; Inf; Inf; Inf]
  Grid_op_CCVSC.op_report.States_(5) = opcond.StateReport
  Grid_op_CCVSC.op_report.States_(5).dx_ = [-8.42021724855e-19; -1.03750341651e-11; 1.8066117432e-12; -2.1979271736e-08; -3.14934577617e-12; -1.28780199837e-07; -3.59431151509e-09; -9.4528940231e-10; 1.95485394618e-11; 3.47507380102e-10; -9.08167885259e-11]
  Grid_op_CCVSC.op_report.States_(5).Nx_ = 11
  Grid_op_CCVSC.op_report.States_(5).Block_ = 'untitled/CCVSC/P'
  Grid_op_CCVSC.op_report.States_(5).x_ = [1.01727038409e-18; 0.400000000001; -1.80456749167e-13; 4.5000000022; 3.15175961175e-13; 3.10000001288; 2.32400000036; 0.400000000095; -1.95503794004e-12; -3.47571023681e-11; 9.07830100881e-12]
  Grid_op_CCVSC.op_report.States_(5).SteadyState_ = [1; 1; 1; 1; 1; 1; 1; 1; 1; 1; 1]
  Grid_op_CCVSC.op_report.States_(5).dxMin_ = [-Inf; -Inf; -Inf; -Inf; -Inf; -Inf; -Inf; -Inf; -Inf; -Inf; -Inf]
  Grid_op_CCVSC.op_report.States_(5).dxMax_ = [Inf; Inf; Inf; Inf; Inf; Inf; Inf; Inf; Inf; Inf; Inf]
  Grid_op_CCVSC.op_report.States_(5).Known_ = [0; 0; 0; 0; 0; 0; 0; 0; 0; 0; 0]
  Grid_op_CCVSC.op_report.States_(5).Min_ = [-Inf; -Inf; -Inf; -Inf; -Inf; -Inf; -Inf; -Inf; -Inf; -Inf; -Inf]
  Grid_op_CCVSC.op_report.States_(5).Max_ = [Inf; Inf; Inf; Inf; Inf; Inf; Inf; Inf; Inf; Inf; Inf]
  Grid_op_CCVSC.op_report.States_(6) = opcond.StateReport
  Grid_op_CCVSC.op_report.States_(6).dx_ = [0; 2.68729483111e-12; 3.79418718666e-12; 8.72443783884e-11; 4.44810854816e-12; 3.83996723308e-10; 1.44183276429e-12; 5.59829960167e-13; 7.40518757425e-13; -1.09456887998e-11; -1.15710219184e-11]
  Grid_op_CCVSC.op_report.States_(6).Nx_ = 11
  Grid_op_CCVSC.op_report.States_(6).Block_ = 'untitled/CCVSC/PLL/dynamic/PLL/I'
  Grid_op_CCVSC.op_report.States_(6).x_ = [1; 1; 1; 0.999999999991; 1; 0.999999999962; 1; 1; 1; 1; 1]
  Grid_op_CCVSC.op_report.States_(6).SteadyState_ = [1; 1; 1; 1; 1; 1; 1; 1; 1; 1; 1]
  Grid_op_CCVSC.op_report.States_(6).dxMin_ = [-Inf; -Inf; -Inf; -Inf; -Inf; -Inf; -Inf; -Inf; -Inf; -Inf; -Inf]
  Grid_op_CCVSC.op_report.States_(6).dxMax_ = [Inf; Inf; Inf; Inf; Inf; Inf; Inf; Inf; Inf; Inf; Inf]
  Grid_op_CCVSC.op_report.States_(6).Known_ = [0; 0; 0; 0; 0; 0; 0; 0; 0; 0; 0]
  Grid_op_CCVSC.op_report.States_(6).Min_ = [-Inf; -Inf; -Inf; -Inf; -Inf; -Inf; -Inf; -Inf; -Inf; -Inf; -Inf]
  Grid_op_CCVSC.op_report.States_(6).Max_ = [Inf; Inf; Inf; Inf; Inf; Inf; Inf; Inf; Inf; Inf; Inf]
  Grid_op_CCVSC.op_report.States_(7) = opcond.StateReport
  Grid_op_CCVSC.op_report.States_(7).dx_ = [0; 0; 0; 0; 6.97573699602e-14; 9.13821546478e-12; 6.97573699602e-14; 6.97573699602e-14; 0; 1.11611791936e-12; -4.18544219761e-13]
  Grid_op_CCVSC.op_report.States_(7).Nx_ = 11
  Grid_op_CCVSC.op_report.States_(7).Block_ = 'untitled/CCVSC/PLL/dynamic/frame'
  Grid_op_CCVSC.op_report.States_(7).x_ = [-0.0165344013704; -0.0868074935304; -0.132939939029; -0.0594865631615; -0.148813342999; -0.166175316605; 0.0365926525094; -0.0554181853462; -0.184088222665; -0.199439311658; -0.180945834503]
  Grid_op_CCVSC.op_report.States_(7).SteadyState_ = [1; 1; 1; 1; 1; 1; 1; 1; 1; 1; 1]
  Grid_op_CCVSC.op_report.States_(7).dxMin_ = [-Inf; -Inf; -Inf; -Inf; -Inf; -Inf; -Inf; -Inf; -Inf; -Inf; -Inf]
  Grid_op_CCVSC.op_report.States_(7).dxMax_ = [Inf; Inf; Inf; Inf; Inf; Inf; Inf; Inf; Inf; Inf; Inf]
  Grid_op_CCVSC.op_report.States_(7).Known_ = [0; 0; 0; 0; 0; 0; 0; 0; 0; 0; 0]
  Grid_op_CCVSC.op_report.States_(7).Min_ = [-Inf; -Inf; -Inf; -Inf; -Inf; -Inf; -Inf; -Inf; -Inf; -Inf; -Inf]
  Grid_op_CCVSC.op_report.States_(7).Max_ = [Inf; Inf; Inf; Inf; Inf; Inf; Inf; Inf; Inf; Inf; Inf]
  Grid_op_CCVSC.op_report.States_(8) = opcond.StateReport
  Grid_op_CCVSC.op_report.States_(8).dx_ = [-3.46944695195e-17; -6.46714626296e-11; -7.22963355848e-12; -8.82571127292e-09; -7.94676824345e-12; -5.54142687292e-08; -2.61821259118e-10; -4.6777914875e-10; -1.31483157695e-10; -9.21122622621e-10; -2.07436290367e-10]
  Grid_op_CCVSC.op_report.States_(8).Nx_ = 11
  Grid_op_CCVSC.op_report.States_(8).Block_ = 'untitled/CCVSC/Q'
  Grid_op_CCVSC.op_report.States_(8).x_ = [-0.015862822257; 0.120252486258; 0.0522438711347; 0.647307088531; 0.0546742450618; 1.36800880468; -0.0931237077542; 1.06159295924; 0.342624354062; 0.31755952052; 0.276277445204]
  Grid_op_CCVSC.op_report.States_(8).SteadyState_ = [1; 1; 1; 1; 1; 1; 1; 1; 1; 1; 1]
  Grid_op_CCVSC.op_report.States_(8).dxMin_ = [-Inf; -Inf; -Inf; -Inf; -Inf; -Inf; -Inf; -Inf; -Inf; -Inf; -Inf]
  Grid_op_CCVSC.op_report.States_(8).dxMax_ = [Inf; Inf; Inf; Inf; Inf; Inf; Inf; Inf; Inf; Inf; Inf]
  Grid_op_CCVSC.op_report.States_(8).Known_ = [0; 0; 0; 0; 0; 0; 0; 0; 0; 0; 0]
  Grid_op_CCVSC.op_report.States_(8).Min_ = [-Inf; -Inf; -Inf; -Inf; -Inf; -Inf; -Inf; -Inf; -Inf; -Inf; -Inf]
  Grid_op_CCVSC.op_report.States_(8).Max_ = [Inf; Inf; Inf; Inf; Inf; Inf; Inf; Inf; Inf; Inf; Inf]
  Grid_op_IG : object (value not decoded)
  Grid_op_MGES : object (value not decoded)
  Grid_op_SG : object (value not decoded)
  Grid_op_VSM : object (value not decoded)
  Grid_shift_lines = [0 0 0 0]
  Grid_tap_lines = [1 1 1 1]
  Grid_v_buses_mod = [1 1 1 0.9837920967 1]
  LinsysParamChangeStruct : Param1 (value not decoded)
  Lline = 0.01
  Rline = 1e-05
  linsys = ss
  linsys.InputName_ = "Assignment1(1,1)"
  linsys.OutputName_ = "Selector7/f(1)"
  linsys.IOSize_ = [1 1]
  linsys.Data_ = ltipack.ssdata
  linsys.Data_.StateName : string (value not decoded)
  linsys.Data_.StatePath : string (value not decoded)
  linsys.Data_.a = [-100 0 0 0 0 0 0 0 0 0 0 0 ... (473344 elements, 688x688)]
  linsys.Data_.b = [0 0 0 0 0 0 0 0 0 0 0 0 ... (688 elements, 688x1)]
  linsys.Data_.c = [-0.001 0 0 0 0 0 0 0 0 0 0 0 0 0 0 0 0 0 0 0 0 0 0 0 0 0 0 0 0 0 0 0 0 0 0 0 0 0 0 0 0 0 0 0 0 0 0 0 0 0 0 0 0 0 0 0 0 0 0 0 0 0 0 0 0 0 0 0 0 0 0 0 0 0 0 0 0 0 0 0 0 0 0 0 0 0 0 0 0 0 0 0 0 0 0 0 0 0 0 0 0 0 0 0 0 0 0 0 0 0 0 0 0 0 0 0 0 0 0 0 0 0 0 0 0 0 0 0 0 0 0 0 0 0 0 0 0 0 0 0 0 0 0 0 0 0 0 0 0 0 0 0 0 0 0 0 0 0 0 0 0 0 0 0 0 0 0 0 0 0 0 0 0 0 0 0 0 0 0 0 0 0 0 0 0 0 0 0 0 0 0 0 0 0 0 0 0 0 0 0 0 0 0 0 0 0 0 0 0 0 0 0 0 0 0 0 0 0 0 0 0 0 0 0 0 0 0 0 0 0 0 0 0 0 0 0 0 0 0 0 0 0 0 0 0 0 0 0 0 0 0 0 0 0 0 0 0 0 0 0 0 0 0 0 0 0 0 0 0 0 0 0 0 0 0 0 0 0 0 0 0 0 0 0 0 0 0 0 0 0 0 0 0 0 0 0 0 0 0 0 0 0 0 0 0 0 0 0 0 0 0 0 0 0 0 0 0 0 0 0 0 0 0 0 0 0 0 0 0 0 0 0 0 0 0 0 0 0 0 0 0 0 0 0 0 0 0 0 0 0 0 0 0 0 0 0 0 0 0 0 0 0 0 0 0 0 0 0 0 0 0 0 0 0 0 0 0 0 0 0 0 0 0 0 0 0 0 0 0 0 0 0 0 0 0 0 0 0 0 0 0 0 0 0 0 0 0 0 0 0 0 0 0 0 0 0 0 0 0 0 0 0 0 0 0 0 0 0 0 0 0 0 0 0 0 0 0 0 0 0 0 0 0 0 0 0 0 0 0 0 0 0 0 0 0 0 0 0 0 0 0 0 0 0 0 0 0 0 0 0 0 0 0 0 0 0 0 0 0 0 0 0 0 0 0 0 0 0 0 0 0 0 0 0 0 0 0 0 0 0 0 0 0 0 0 0 0 0 0 0 0 0 0 0 0 0 0 0 0 0 0 0 0 0 0 0 0 0 0 0 0 0 0 0 0 0 0 0 0 0 0 0 0 0 0 0 0 0 0 0 0 0 0 0 0 0 0 0 0 0 0 0 0 0 0 0 0 0 0 0 0 0 0 0 0 0 0 0 0 0 0 0 0 0 0 0 0 0 0 0 0 0 0 0 0 0 0 0 0 0 0 0 0 0 0 0 0 0 0 0 0 0 0 0 0 0 0 0 0 0 0 0 0 0 0 0 0 0 0 0 0 0 0 0 0 0 0 0 0 0 0 0 0 0 0 0 0 0 0 0 0 0 0 0 0 0 0 0 0 0 0 0 0 0 0 0 0 0 0 0 0 0 0 0 0 0 0 0 0 0 0 0 0 0 0 0 0 0]
  linsys.Data_.d = 0
  linsys.Data_.dx0 = [0 0 0 0 0 0 0 0 0 0 0 0 ... (688 elements, 688x1)]
  linsys.Data_.x0 = [0 0 0 0 0 0 0 0 0 0 0 0 ... (688 elements, 688x1)]
  linsys.Data_.u0 = 0
  linsys.Data_.y0 = 0
  linsys.Data_.Delay.Input = 0
  linsys.Data_.Delay.Output = 0
  linsys.Data_.Delay.Internal = []
  linsys.Data_.Ts = 0
symbols that are objects in the model workspace (value not decoded): Grid_op_IG, Grid_op_MGES, Grid_op_SG, Grid_op_VSM
undefined symbols (not defined in the file): block_buses_DC, block_idx, CCVSC_idx, Cf, costs, costs2, D, DFIGs_nodes, DiscIntNeverNeededParam, entity, Fb, Fi, From_nodes, grid_linsys, Grid_op_DFIG, Grid_op_DFIG_PQ, Grid_op_MSG, Grid_op_SC, Grid_op_VCVSC, H, initial_states_grid, K_1, K_3, K_5, K_A, K_C, K_IM, K_IR, K_P, K_PM, K_PR, K_S1, K_S2, K_S3, Ki_w, Kic, Kiv, Kp_id, Kp_theta, Kp_w, Kpc, Kpv, last_send, Lc, Lf, Lfd, Lkd1, Lkd2, Lkq1, Lkq2, Lkq3, Lmd, Lmq, Lsd, Lsq, m, M, Matrix_flux_to_i, mp, MSGs_buses ... (+44)
libraries: simulink x1048, eeGeneralControl x12
(part 2 of 50)

== system VFlexP/Grid/DCAC converters ==
  note: mdlWks = get_param(bdroot,'ModelWorkspace'); % Get the model workspace
      | block_name = get_param(gcb,'Name');
      | bvarname = get_param(get_param(get_param(get_param(...
      | gcb, 'Parent'), 'Parent'), 'Parent'), 'bvarname');
      | DC = mdlWks.getVariable([bvarname 'DC']);
      | try
      | block_DC_buses = DC.(block_name + "s_DC_buses");
      | block_buses = DC.(block_name + "s_buses");
      | block_DC_toM = DC.(block_name + "s_DC_toM");
      | block_toM = DC.(block_name + "s_toM");
      | dparams = DC.(block_name + "_dparams");
      | fref = mdlWks.getVariable([bvarname 'fref']);
      | block_fref = fref.(block_name);
      | catch ME
      | errordlg(ME.message)
      | end
  vac : Inport
  vdc : Inport  Port=2
  DC_CCVSC : Subsystem  mask(CCVSC){Pmax=0, Qmax=0, fb=50, dynamic_CC=Dynamic, Tint=0.1, Kint=1, Bint=1, dynamic_PLL=Dynamic, kpi=1, kii=10, Tf=0.01, alphapcoef=0, alphaqcoef=0, Prel=1, Qrel=1, Eref=1, kp=10, kq=10}
      mask prompts: Pmax "Active power limit (p.u.)"; Qmax "Reactive power limit (p.u.)"; fb "Base frequency (Hz)"; dynamic_CC "Dynamic behaviour"; dynamic_PLL "Dynamic behaviour"; Tf "LPF time constant (s)"; alphapcoef "P droop coefficient"; alphaqcoef "Q droop coefficient"; Prel "P/P_NmP"; Qrel "Q/Q_NnQ"; Eref "Nominal voltage of PCC"; kp "P gain"; kq "Q gain"
      mask help: Grid-following converter. CC is the current controller. Dynamic behavior includes the PI controller, decoupling and output inductance. Static behavior consists of setting the reference current directly in the output. PC is the power controller including the current reference calculation and low-pass filters for the power measurements.
      mask init:
      | mdlWks = get_param(bdroot,'ModelWorkspace'); % Get the model workspace
      | block_name = get_param(gcb,'Name');
      | bvarname = get_param(get_param(get_param(get_param(...
      |         gcb, 'Parent'), 'Parent'), 'Parent'), 'bvarname');
      | DC = mdlWks.getVariable([bvarname 'DC']);
      | try
      |     block_DC_buses = DC.(block_name + "s_DC_buses");
      |     block_buses = DC.(block_name + "s_buses");
      |     block_DC_toM = DC.(block_name + "s_DC_toM");
      |     block_toM = DC.(block_name + "s_toM");
      |     dparams = DC.(block_name + "_dparams");
      |     fref = mdlWks.getVariable([bvarname 'fref']);
      |     block_fref = fref.(block_name);
      | catch ME
      |     %errordlg(ME.message) 
      | end
      | 
      | 
      | block = gcb;
      | if Tf ~= 0
      |     iTf = 1/Tf;
      |     set_param([block '/PC/LPF_d'],'Commented','off')
      |     set_param([block '/PC/LPF_q'],'Commented','off')
      |     set_param([block '/LPF_d'],'Commented','off')
      |     set_param([block '/LPF_q'],'Commented','off')
      | else
      |     set_param([block '/PC/LPF_d'],'Commented','through')
      |     set_param([block '/PC/LPF_q'],'Commented','through')
      |     set_param([block '/LPF_d'],'Commented','through')
      |     set_param([block '/LPF_q'],'Commented','through')
      | end
      mask Help: web('Documentation/CCVSC.html')
      mask TypeOptions dynamic_CC: Dynamic | Static
      mask Callback dynamic_CC:
      | block = gcb;
      | dynamic = get_param(block, 'dynamic_CC');
      | param_vis = get_param(block,'MaskVisibilities');
      | block_params = string(fieldnames(get_param(block, 'DialogParameters')));
      | switch dynamic
      |     case 'Dynamic'
      |         set_param([gcb '/CC'], 'LabelModeActiveChoice', 'dynamic')
      |         param_vis(find(block_params == 'Tint'):find(block_params == 'Rf')) = cellstr("on");
      |     case 'Static'
      |         set_param([gcb '/CC'], 'LabelModeActiveChoice', 'static')
      |         param_vis(find(block_params == 'Tint'):find(block_params == 'Rf')) = cellstr("off");
      | end
      | set_param(block,'MaskVisibilities',param_vis)
      mask TypeOptions dynamic_PLL: Dynamic | Static
      mask Callback dynamic_PLL:
      | block = gcb;
      | dynamic = get_param(block, 'dynamic_PLL');
      | param_vis = get_param(block,'MaskVisibilities');
      | block_params = string(fieldnames(get_param(block, 'DialogParameters')));
      | switch dynamic
      |     case 'Dynamic'
      |         set_param([gcb '/PLL'], 'LabelModeActiveChoice', 'dynamic')
      |         param_vis(find(block_params == 'kpi'):find(block_params == 'kii')) = cellstr("on");
      |     case 'Static'
      |         set_param([gcb '/PLL'], 'LabelModeActiveChoice', 'static')
      |         param_vis(find(block_params == 'kpi'):find(block_params == 'kii')) = cellstr("off");
      | end
      | set_param(block,'MaskVisibilities',param_vis)
      mask DialogControl CC Prompt: CC
      mask DialogControl PLL Prompt: PLL
      mask DialogControl PC Prompt: PC
      mask DialogControl SC Prompt: SC
  DC_VCVSC : Subsystem  Commented=on  mask(VCVSC){Pmax=Inf, Qmax=Inf, fb=50, dynamic_VCC=Static, Lf=0.01, Rf=0.001, Rcf=1000000, Cfi=0.1, Kint=1, Tint=0.1, Bint=1, Kext=1, Bext=1, Text=0.1, Fi=1, Tf=0.01, mp=0.01, nq=0.01, VI_L=0.1, VI_R=0.01, WOF_Tf=0, cf=0.1, cv=0.1, L_out=0.1, R_out=0.01}
      mask prompts: Pmax "Active power limit (p.u.)"; Qmax "Reactive power limit (p.u.)"; fb "Base frequency (Hz)"; dynamic_VCC "Dynamic behavior"; Lf "Filter inductance (pu)"; Rf "Filter resistance (pu)"; Rcf "Parallel resistance to C (pu)"; Cfi "Filter capacitance (pu)"; Fi "Current feedfordward gain"; Tf "Low-pass filter time constant (s)"; mp "Droop coefficient mp (pu)"; nq "Droop coefficient nq (pu)"; VI_L "Inductance (pu)"; VI_R "Resistance (pu)"; WOF_Tf "WOF time constant (s)"; cf "Frequency SC gain"; cv "Voltage SC gain"; L_out "Output inductance (p.u.)"; R_out "Output resistance (p.u.)"
      mask help: Grid-forming converter. VCC are the voltage and current controllers. Dynamic behavior includes the PI controllers, decoupling, current feedfordward and LC output filter. Static behavior consists of setting the reference voltage directly in the output. PC is the power controller including the droop control and low-pass filters for the power measurements.
      mask init:
      | mdlWks = get_param(bdroot,'ModelWorkspace'); % Get the model workspace
      | block_name = get_param(gcb,'Name');
      | bvarname = get_param(get_param(get_param(get_param(...
      |         gcb, 'Parent'), 'Parent'), 'Parent'), 'bvarname');
      | DC = mdlWks.getVariable([bvarname 'DC']);
      | try
      |     block_DC_buses = DC.(block_name + "s_DC_buses");
      |     block_buses = DC.(block_name + "s_buses");
      |     block_DC_toM = DC.(block_name + "s_DC_toM");
      |     block_toM = DC.(block_name + "s_toM");
      |     dparams = DC.(block_name + "_dparams");
      | catch ME
      |     %errordlg(ME.message)
      | end
      mask Help: web('Documentation/VCVSC.html')
      mask TypeOptions dynamic_VCC: Dynamic with limitation | Dynamic | Static | Dynamic VC and static CC
      mask Callback dynamic_VCC:
      | block = gcb;
      | dynamic = get_param(block, 'dynamic_VCC');
      | param_vis = get_param(block,'MaskVisibilities');
      | block_params = string(fieldnames(get_param(block, 'DialogParameters')));
      | switch dynamic
      |     case 'Dynamic'
      |         param_vis(find(block_params == 'Lf'):find(block_params == 'Fi')) = cellstr("on");
      |         set_param([gcb '/VCC'], 'LabelModeActiveChoice', 'dynamic');
      |     case 'Dynamic with limitation'
      |         param_vis(find(block_params == 'Lf'):find(block_params == 'Fi')) = cellstr("on");
      |         set_param([gcb '/VCC'], 'LabelModeActiveChoice', 'dynamic_limiting');
      |     case 'Static'
      |         param_vis(find(block_params == 'Lf'):find(block_params == 'Fi')) = cellstr("off");
      |         set_param([gcb '/VCC'], 'LabelModeActiveChoice', 'static');
      |     case 'Dynamic VC and static CC'
      |         param_vis(find(block_params == 'Lf'):find(block_params == 'Fi')) = cellstr("on");
      |         param_vis(ismember(block_params, ["Lf","Rf","Kpc","Kic","Fi"])) = cellstr("off");
      |         set_param([gcb '/VCC'], 'LabelModeActiveChoice', 'dynamic_VC');
      | end
      | set_param(block,'MaskVisibilities',param_vis)
      mask TypeOptions Tf: PC/Tf
      mask TypeOptions mp: PC/mp
      mask TypeOptions nq: PC/nq
      mask TypeOptions VI_L: VI/L
      mask TypeOptions VI_R: VI/R
      mask TypeOptions WOF_Tf: VI/Tf
      mask DialogControl Container8 Prompt: Parameters
      mask DialogControl VCC Prompt: VCC
      mask DialogControl PC Prompt: PC
      mask DialogControl VI Prompt: VI
      mask DialogControl SC Prompt: SC
      mask DialogControl Container9 Prompt: Others
  DC_VSM : Subsystem  Commented=on  mask(VCVSC){Pmax=Inf, Qmax=Inf, fb=50, dynamic_VCC=Dynamic with P limitation, Lf=Lf, Rf=Rf, Rcf=1000000, Cfi=Cf, Kint=Kpc, Tint=Kpc/Kic, Bint=1, Kext=Kpv, Bext=1, Text=Kpv/Kiv, Fi=Fi, Hv=Tf/(2*mp), Dv=0, Rv=mp, nq=nq, VI_L=VI_L, VI_R=VI_R, WOF_Tf=WOF_Tf, cf=0.1, cv=0.1, L_out=Lc, R_out=Rc}
      mask prompts: Pmax "Active power limit (p.u.)"; Qmax "Reactive power limit (p.u.)"; fb "Base frequency (Hz)"; dynamic_VCC "Dynamic behavior"; Lf "Filter inductance (pu)"; Rf "Filter resistance (pu)"; Rcf "Parallel resistance to C (pu)"; Cfi "Filter capacitance (pu)"; Fi "Current feedfordward gain"; Hv "Inertia"; Dv "Damping"; Rv "Droop Rv"; nq "Droop nq"; VI_L "Inductance (pu)"; VI_R "Resistance (pu)"; WOF_Tf "WOF time constant (s)"; cf "Frequency SC gain"; cv "Voltage SC gain"; L_out "Output inductance (p.u.)"; R_out "Output resistance (p.u.)"
      mask help: Grid-forming converter. VCC are the voltage and current controllers. Dynamic behavior includes the PI controllers, decoupling, current feedfordward and LC output filter. Static behavior consists of setting the reference voltage directly in the output. PC is the power controller including the droop control and low-pass filters for the power measurements.
      mask init:
      | mdlWks = get_param(bdroot,'ModelWorkspace'); % Get the model workspace
      | block_name = get_param(gcb,'Name');
      | bvarname = get_param(get_param(get_param(get_param(...
      |         gcb, 'Parent'), 'Parent'), 'Parent'), 'bvarname');
      | DC = mdlWks.getVariable([bvarname 'DC']);
      | try
      |     block_DC_buses = DC.(block_name + "s_DC_buses");
      |     block_buses = DC.(block_name + "s_buses");
      |     block_DC_toM = DC.(block_name + "s_DC_toM");
      |     block_toM = DC.(block_name + "s_toM");
      |     dparams = DC.(block_name + "_dparams");
      |     fref = mdlWks.getVariable([bvarname 'fref']);
      |     block_fref = fref.(block_name);
      | catch ME
      |     %errordlg(ME.message) 
      | end
      mask Help: web('Documentation/VCVSC.html')
      mask TypeOptions dynamic_VCC: Dynamic with limitation | Dynamic with P limitation | Dynamic | Static | Dynamic VC and static CC
      mask Callback dynamic_VCC:
      | block = gcb;
      | dynamic = get_param(block, 'dynamic_VCC');
      | param_vis = get_param(block,'MaskVisibilities');
      | block_params = string(fieldnames(get_param(block, 'DialogParameters')));
      | switch dynamic
      |     case 'Dynamic'
      |         param_vis(find(block_params == 'Lf'):find(block_params == 'Fi')) = cellstr("on");
      |         set_param([gcb '/VCC'], 'LabelModeActiveChoice', 'dynamic');
      |     case 'Dynamic with limitation'
      |         param_vis(find(block_params == 'Lf'):find(block_params == 'Fi')) = cellstr("on");
      |         set_param([gcb '/VCC'], 'LabelModeActiveChoice', 'dynamic_limiting');
      |     case 'Dynamic with P limitation'
      |         param_vis(find(block_params == 'Lf'):find(block_params == 'Fi')) = cellstr("on");
      |         set_param([gcb '/VCC'], 'LabelModeActiveChoice', 'dynamic_limiting_P');
      |     case 'Static'
      |         param_vis(find(block_params == 'Lf'):find(block_params == 'Fi')) = cellstr("off");
      |         set_param([gcb '/VCC'], 'LabelModeActiveChoice', 'static');
      |     case 'Dynamic VC and static CC'
      |         param_vis(find(block_params == 'Lf'):find(block_params == 'Fi')) = cellstr("on");
      |         param_vis(ismember(block_params, ["Lf","Rf","Kpc","Kic","Fi"])) = cellstr("off");
      |         set_param([gcb '/VCC'], 'LabelModeActiveChoice', 'dynamic_VC');
      | end
      | set_param(block,'MaskVisibilities',param_vis)
      mask TypeOptions VI_L: VI/L
      mask TypeOptions VI_R: VI/R
      mask TypeOptions WOF_Tf: VI/Tf
      mask DialogControl Container8 Prompt: Parameters
      mask DialogControl VCC Prompt: VCC
      mask DialogControl PC Prompt: PC
      mask DialogControl VI Prompt: VI
      mask DialogControl SC Prompt: SC
      mask DialogControl Container9 Prompt: Others
  Sum : Sum  Inputs=|+++
  Sum1 : Sum  Inputs=|+++
  iac : Outport
  idc : Outport  Port=2
  wires:
  [vac] -> DC_CCVSC/1(vac)
  [vac] -> DC_VCVSC/1(vac)
  vac/1 -> [vac]
  DC_VCVSC/1(iac) -> Sum/1
  Sum/1 -> iac/1
  DC_CCVSC/1(iac) -> Sum/2
  [vdc] -> DC_VCVSC/2(vdc)
  DC_VCVSC/2(idc) -> Sum1/1
  Sum1/1 -> idc/1
  DC_CCVSC/2(idc) -> Sum1/2
  [vdc] -> DC_CCVSC/2(vdc)
  vdc/1 -> [vdc]
  [vdc] -> DC_VSM/2(vdc)
  [vac] -> DC_VSM/1(vac)
  DC_VSM/2(idc) -> Sum1/3
  DC_VSM/1(iac) -> Sum/3
